simulink model "qinit"  (Simulink 7.9)
settings: Solver=ode45  StartTime=0.0  StopTime=10.0  RelTol=1e-3
settings Model: Creator=jorhabib  LastModifiedBy=jorhabib

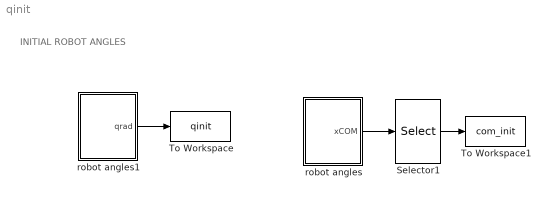
== system qinit ==
  note: INITIAL ROBOT ANGLES
  Selector1 : Selector  IndexMode=Zero-based  InputPortWidth=7  IndexOptions=Index vector (dialog)  Indices=[0:1]  OutputSizes=1
  To Workspace : ToWorkspace  VariableName=qinit  SampleTime=-1
  To Workspace1 : ToWorkspace  VariableName=com_init  SampleTime=-1
  robot angles : Subsystem
  robot angles1 : Subsystem
  wires:
  robot angles1/1(qrad) -> To Workspace/1
  robot angles/1(xCOM) -> Selector1/1
  Selector1/1 -> To Workspace1/1

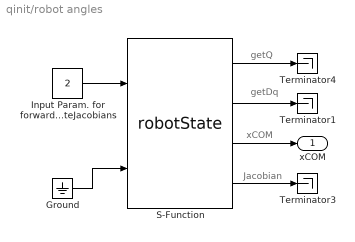
== system qinit/robot angles ==
  note: getDq
  note: xCOM
  note: getQ
  note: Jacobian
  Ground : Ground
  "Input Param. for forwardKinematics and  computeJacobians " : Constant  Value=2  OutDataTypeStr=int8
  S-Function : S-Function  FunctionName=robotState  Parameters=val,robotname,localname  EnableBusSupport=off  mask{val=2, robotname='icubSim', localname='robotState'}
      mask prompts: val "Value"; robotname "Robot Name (icub - icubSim)"; localname "Module Name"
  Terminator1 : Terminator
  Terminator3 : Terminator
  Terminator4 : Terminator
  xCOM : Outport
  wires:
  Ground/1 -> S-Function/2
  S-Function/2 -> Terminator1/1
  S-Function/1 -> Terminator4/1
  S-Function/3 -> xCOM/1
  "Input Param. for forwardKinematics and  computeJacobians "/1 -> S-Function/1
  S-Function/4 -> Terminator3/1

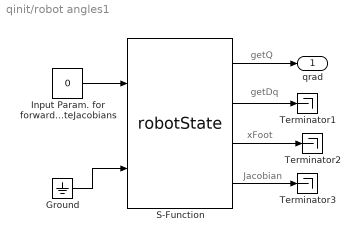
== system qinit/robot angles1 ==
  note: Jacobian
  note: getQ
  note: xFoot
  note: getDq
  Ground : Ground
  "Input Param. for forwardKinematics and  computeJacobians " : Constant  Value=0  OutDataTypeStr=int8
  S-Function : S-Function  FunctionName=robotState  Parameters=val,robotname,localname  EnableBusSupport=off  mask{val=0, robotname='icubSim', localname='robotState'}
      mask prompts: val "Value"; robotname "Robot Name (icub - icubSim)"; localname "Module Name"
  Terminator1 : Terminator
  Terminator2 : Terminator
  Terminator3 : Terminator
  qrad : Outport
  wires:
  S-Function/4 -> Terminator3/1
  "Input Param. for forwardKinematics and  computeJacobians "/1 -> S-Function/1
  S-Function/3 -> Terminator2/1
  S-Function/1 -> qrad/1
  S-Function/2 -> Terminator1/1
  Ground/1 -> S-Function/2
